simulink model "scheme_2"  (R2017a)
settings: Solver=VariableStepAuto  StartTime=0.0  StopTime=10.0  RelTol=1e-3
libraries: simulink x3
settings Model: Creator=igorkislyuk  LastModifiedBy=igorkislyuk

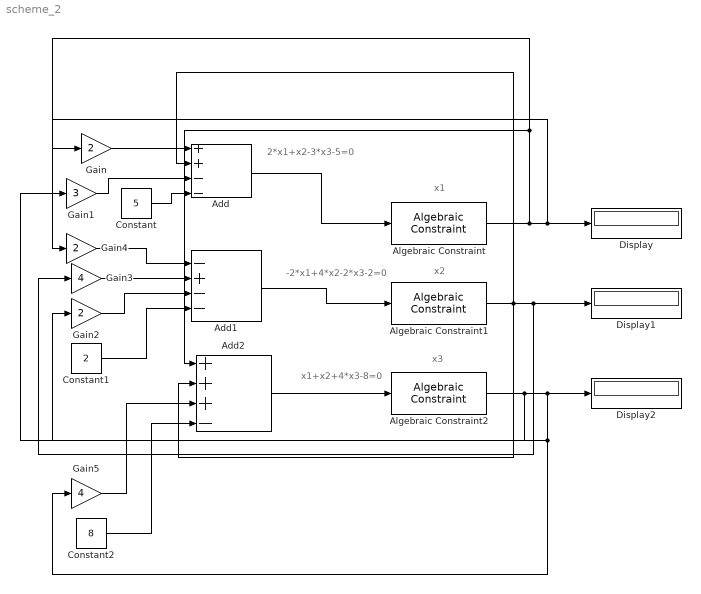
== system scheme_2 ==
  note: x1+x2+4*x3-8=0
  note: -2*x1+4*x2-2*x3-2=0
  note: 2*x1+x2-3*x3-5=0
  note: x3
  note: x2
  note: x1
  Add : Sum  Inputs=++--
  Add1 : Sum  Inputs=-+--
  Add2 : Sum  Inputs=+++-
  Algebraic Constraint : simulink/Math Operations/Algebraic Constraint  z0=3
      settings: SourceProductName=Simulink  SourceProductBaseCode=SL
  Algebraic Constraint1 : simulink/Math Operations/Algebraic Constraint  z0=3
      settings: SourceProductName=Simulink  SourceProductBaseCode=SL
  Algebraic Constraint2 : simulink/Math Operations/Algebraic Constraint  z0=3
      settings: SourceProductName=Simulink  SourceProductBaseCode=SL
  Constant : Constant  Value=5
  Constant1 : Constant  Value=2
  Constant2 : Constant  Value=8
  Display : Display
  Display1 : Display
  Display2 : Display
  Gain : Gain  Gain=2
  Gain1 : Gain  Gain=3
  Gain2 : Gain  Gain=2
  Gain3 : Gain  Gain=4
  Gain4 : Gain  Gain=2
  Gain5 : Gain  Gain=4
  wires:
  Algebraic Constraint1/1 -> Add2/2, Add/2, Gain3/1, Display1/1
  Algebraic Constraint2/1 -> Gain1/1, Gain5/1, Gain2/1, Display2/1
  Add/1 -> Algebraic Constraint/1
  Gain/1 -> Add/1
  Algebraic Constraint/1 -> Add2/1, Gain/1, Gain4/1, Display/1
  Gain1/1 -> Add/3
  Constant/1 -> Add/4
  Add1/1 -> Algebraic Constraint1/1
  Constant1/1 -> Add1/4
  Gain2/1 -> Add1/3
  Gain3/1 -> Add1/2
  Gain4/1 -> Add1/1
  Add2/1 -> Algebraic Constraint2/1
  Constant2/1 -> Add2/4
  Gain5/1 -> Add2/3
